simulink model "chibiOS_Config_Test_PAL"  (R2015b)
settings: Solver=FixedStepDiscrete  SolverMode=MultiTasking  StartTime=0.0  StopTime=10.0  RelTol=1e-3
undefined symbols (not defined in the file or in its folder): chSysHalt, STM32_DMA_STREAM_ID
libraries: lib_ChibiOS x3
settings Model: Creator=freyjed  LastModifiedBy=C3038028
settings DataIOCC: LimitDataPoints=off  SaveFormat=Array  SaveOutput=off  SignalLogging=off  DSMLogging=off  SaveTime=off
settings OptimizationCC: BlockReduction=off  ConditionallyExecuteInputs=off  BufferReuse=off  ExpressionDepthLimit=2147483647  OptimizeModelRefInitCode=on  LifeSpan=1
settings DebuggingCC: UnderspecifiedInitializationDetection=Classic  MergeDetectMultiDrivingBlocksExec=none  SolverPrmCheckMsg=warning  StateNameClashWarn=warning
settings HardwareCC: ProdBitPerPointer=32  ProdLargestAtomicInteger=Integer  ProdWordSize=32  ProdHWDeviceType=STMicroelectronics->STM32F4xx 32-bit Cortex-M4  TargetLargestAtomicInteger=Integer  TargetLargestAtomicFloat=Float  TargetIntDivRoundTo=Zero  TargetEndianess=LittleEndian  TargetHWDeviceType=ChibiOS->ChibiOS
settings ModelReferenceCC: UpdateModelReferenceTargets=Force
settings RTWCC: SystemTargetFile=ChibiOS.tlc  GenCodeOnly=on  TemplateMakefile=ChibiOS.tmf  Description=ChibiOS/RT (Embedded RTOS Target)  RetainRTWFile=on  IncludeHyperlinkInReport=on
settings CodeAppCC: ForceParamTrailComments=on  IgnoreCustomStorageClasses=off  OperatorAnnotations=on  SimulinkDataObjDesc=on  SFDataObjDesc=on  MATLABFcnDesc=on  CustomSymbolStrType=$N$R$M  DefineNamingRule=UpperCase  InsertBlockDesc=on  MATLABSourceComments=on  InternalIdentifier=Classic  ReqsInCode=on
settings STFCustomTargetCC: ModelReferenceCompliant=off  ConcurrentExecutionCompliant=off  IncludeMdlTerminateFcn=off  GeneratePreprocessorConditionals=Use local settings  CombineOutputUpdateFcns=on  ERTCustomFileBanners=on  SupportContinuousTime=off  SupportNonInlinedSFcns=off  ParenthesesLevel=Maximum  MATLABClassNameForMDSCustomization=Simulink.SoftwareTarget.ERTCustomization  CPPClassGenCompliant=off  GRTInterface=off  SystemTargetFile=ChibiOS.tlc
settings ERTTargetCC: ModelReferenceCompliant=off  ParMdlRefBuildCompliant=off  CompOptLevelCompliant=off  ConcurrentExecutionCompliant=off  IncludeMdlTerminateFcn=off  ERTFirstTimeCompliant=off  ParenthesesLevel=Maximum  ModelStepFunctionPrototypeControlCompliant=off  CPPClassGenCompliant=off  UseToolchainInfoCompliant=off  ERTSrcFileBannerTemplate=chibiOS_sourceFileTemplate.cgt  ERTHdrFileBannerTemplate=chibiOS_sourceFileTemplate.cgt  ERTDataSrcFileTemplate=chibiOS_sourceFileTemplate.cgt  ERTDataHdrFileTemplate=chibiOS_sourceFileTemplate.cgt  ERTCustomFileTemplate=chibiOS_customRoutineProcess.tlc  PreserveExpressionOrder=on  PreserveIfCondition=on  ConvertIfToSwitch=on
settings ConfigComp: CovModelRefEnable=Off

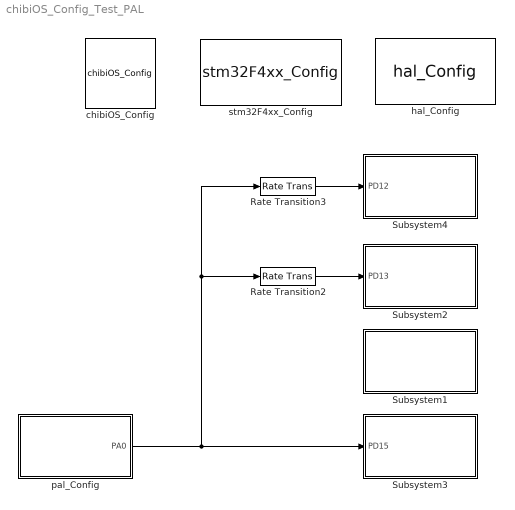
== system chibiOS_Config_Test_PAL ==
  Rate Transition2 : RateTransition
  Rate Transition3 : RateTransition
  Subsystem1 : Subsystem  mask(pal_Config){portName=D, pin0=Disabled, pin1=Disabled, pin2=Disabled, pin3=Disabled, pin4=Disabled, pin5=Disabled, pin6=Disabled, pin7=Disabled, pin8=Disabled, pin9=Disabled, pin10=Disabled, pin11=Disabled, pin12=Disabled, pin13=Disabled, pin14=Toggle, pin15=Disabled, pal_Ts=.9}
      mask prompts: portName "Port"; pin0 "Pin 0"; pin1 "Pin 1"; pin2 "Pin 2"; pin3 "Pin 3"; pin4 "Pin 4"; pin5 "Pin 5"; pin6 "Pin 6"; pin7 "Pin 7"; pin8 "Pin 8"; pin9 "Pin 9"; pin10 "Pin 10"; pin11 "Pin 11"; pin12 "Pin 12"; pin13 "Pin 13"; pin14 "Pin 14"; pin15 "Pin 15"; pal_Ts "Sample Time (-1 for inherited)"
      mask TypeOptions portName: A | B | C | D | E | F | G | H | I
      mask Callback portName: pal_Config_Callback(gcb)
      mask TypeOptions pin0: Disabled | Input - No Pull | Input - Pull Up | Input - Pull Down | Output - Open Drain | Output - Push Pull | Toggle
      mask Callback pin0: pal_Config_Callback(gcb)
      mask TypeOptions pin1: Disabled | Input - No Pull | Input - Pull Up | Input - Pull Down | Output - Open Drain | Output - Push Pull | Toggle
      mask Callback pin1: pal_Config_Callback(gcb)
      mask TypeOptions pin2: Disabled | Input - No Pull | Input - Pull Up | Input - Pull Down | Output - Open Drain | Output - Push Pull | Toggle
      mask Callback pin2: pal_Config_Callback(gcb)
      mask TypeOptions pin3: Disabled | Input - No Pull | Input - Pull Up | Input - Pull Down | Output - Open Drain | Output - Push Pull | Toggle
      mask Callback pin3: pal_Config_Callback(gcb)
      mask TypeOptions pin4: Disabled | Input - No Pull | Input - Pull Up | Input - Pull Down | Output - Open Drain | Output - Push Pull | Toggle
      mask Callback pin4: pal_Config_Callback(gcb)
      mask TypeOptions pin5: Disabled | Input - No Pull | Input - Pull Up | Input - Pull Down | Output - Open Drain | Output - Push Pull | Toggle
      mask Callback pin5: pal_Config_Callback(gcb)
      mask TypeOptions pin6: Disabled | Input - No Pull | Input - Pull Up | Input - Pull Down | Output - Open Drain | Output - Push Pull | Toggle
      mask Callback pin6: pal_Config_Callback(gcb)
      mask TypeOptions pin7: Disabled | Input - No Pull | Input - Pull Up | Input - Pull Down | Output - Open Drain | Output - Push Pull | Toggle
      mask Callback pin7: pal_Config_Callback(gcb)
      mask TypeOptions pin8: Disabled | Input - No Pull | Input - Pull Up | Input - Pull Down | Output - Open Drain | Output - Push Pull | Toggle
      mask Callback pin8: pal_Config_Callback(gcb)
      mask TypeOptions pin9: Disabled | Input - No Pull | Input - Pull Up | Input - Pull Down | Output - Open Drain | Output - Push Pull | Toggle
      mask Callback pin9: pal_Config_Callback(gcb)
      mask TypeOptions pin10: Disabled | Input - No Pull | Input - Pull Up | Input - Pull Down | Output - Open Drain | Output - Push Pull | Toggle
      mask Callback pin10: pal_Config_Callback(gcb)
      mask TypeOptions pin11: Disabled | Input - No Pull | Input - Pull Up | Input - Pull Down | Output - Open Drain | Output - Push Pull | Toggle
      mask Callback pin11: pal_Config_Callback(gcb)
      mask TypeOptions pin12: Disabled | Input - No Pull | Input - Pull Up | Input - Pull Down | Output - Open Drain | Output - Push Pull | Toggle
      mask Callback pin12: pal_Config_Callback(gcb)
      mask TypeOptions pin13: Disabled | Input - No Pull | Input - Pull Up | Input - Pull Down | Output - Open Drain | Output - Push Pull | Toggle
      mask Callback pin13: pal_Config_Callback(gcb)
      mask TypeOptions pin14: Disabled | Input - No Pull | Input - Pull Up | Input - Pull Down | Output - Open Drain | Output - Push Pull | Toggle
      mask Callback pin14: pal_Config_Callback(gcb)
      mask TypeOptions pin15: Disabled | Input - No Pull | Input - Pull Up | Input - Pull Down | Output - Open Drain | Output - Push Pull | Toggle
      mask Callback pin15: pal_Config_Callback(gcb)
  Subsystem2 : Subsystem  mask(pal_Config){portName=D, pin0=Disabled, pin1=Disabled, pin2=Disabled, pin3=Disabled, pin4=Disabled, pin5=Disabled, pin6=Disabled, pin7=Disabled, pin8=Disabled, pin9=Disabled, pin10=Disabled, pin11=Disabled, pin12=Disabled, pin13=Output - Push Pull, pin14=Disabled, pin15=Disabled, pal_Ts=.015*6}
      mask prompts: portName "Port"; pin0 "Pin 0"; pin1 "Pin 1"; pin2 "Pin 2"; pin3 "Pin 3"; pin4 "Pin 4"; pin5 "Pin 5"; pin6 "Pin 6"; pin7 "Pin 7"; pin8 "Pin 8"; pin9 "Pin 9"; pin10 "Pin 10"; pin11 "Pin 11"; pin12 "Pin 12"; pin13 "Pin 13"; pin14 "Pin 14"; pin15 "Pin 15"; pal_Ts "Sample Time (-1 for inherited)"
      mask TypeOptions portName: A | B | C | D | E | F | G | H | I
      mask Callback portName: pal_Config_Callback(gcb)
      mask TypeOptions pin0: Disabled | Input - No Pull | Input - Pull Up | Input - Pull Down | Output - Open Drain | Output - Push Pull | Toggle
      mask Callback pin0: pal_Config_Callback(gcb)
      mask TypeOptions pin1: Disabled | Input - No Pull | Input - Pull Up | Input - Pull Down | Output - Open Drain | Output - Push Pull | Toggle
      mask Callback pin1: pal_Config_Callback(gcb)
      mask TypeOptions pin2: Disabled | Input - No Pull | Input - Pull Up | Input - Pull Down | Output - Open Drain | Output - Push Pull | Toggle
      mask Callback pin2: pal_Config_Callback(gcb)
      mask TypeOptions pin3: Disabled | Input - No Pull | Input - Pull Up | Input - Pull Down | Output - Open Drain | Output - Push Pull | Toggle
      mask Callback pin3: pal_Config_Callback(gcb)
      mask TypeOptions pin4: Disabled | Input - No Pull | Input - Pull Up | Input - Pull Down | Output - Open Drain | Output - Push Pull | Toggle
      mask Callback pin4: pal_Config_Callback(gcb)
      mask TypeOptions pin5: Disabled | Input - No Pull | Input - Pull Up | Input - Pull Down | Output - Open Drain | Output - Push Pull | Toggle
      mask Callback pin5: pal_Config_Callback(gcb)
      mask TypeOptions pin6: Disabled | Input - No Pull | Input - Pull Up | Input - Pull Down | Output - Open Drain | Output - Push Pull | Toggle
      mask Callback pin6: pal_Config_Callback(gcb)
      mask TypeOptions pin7: Disabled | Input - No Pull | Input - Pull Up | Input - Pull Down | Output - Open Drain | Output - Push Pull | Toggle
      mask Callback pin7: pal_Config_Callback(gcb)
      mask TypeOptions pin8: Disabled | Input - No Pull | Input - Pull Up | Input - Pull Down | Output - Open Drain | Output - Push Pull | Toggle
      mask Callback pin8: pal_Config_Callback(gcb)
      mask TypeOptions pin9: Disabled | Input - No Pull | Input - Pull Up | Input - Pull Down | Output - Open Drain | Output - Push Pull | Toggle
      mask Callback pin9: pal_Config_Callback(gcb)
      mask TypeOptions pin10: Disabled | Input - No Pull | Input - Pull Up | Input - Pull Down | Output - Open Drain | Output - Push Pull | Toggle
      mask Callback pin10: pal_Config_Callback(gcb)
      mask TypeOptions pin11: Disabled | Input - No Pull | Input - Pull Up | Input - Pull Down | Output - Open Drain | Output - Push Pull | Toggle
      mask Callback pin11: pal_Config_Callback(gcb)
      mask TypeOptions pin12: Disabled | Input - No Pull | Input - Pull Up | Input - Pull Down | Output - Open Drain | Output - Push Pull | Toggle
      mask Callback pin12: pal_Config_Callback(gcb)
      mask TypeOptions pin13: Disabled | Input - No Pull | Input - Pull Up | Input - Pull Down | Output - Open Drain | Output - Push Pull | Toggle
      mask Callback pin13: pal_Config_Callback(gcb)
      mask TypeOptions pin14: Disabled | Input - No Pull | Input - Pull Up | Input - Pull Down | Output - Open Drain | Output - Push Pull | Toggle
      mask Callback pin14: pal_Config_Callback(gcb)
      mask TypeOptions pin15: Disabled | Input - No Pull | Input - Pull Up | Input - Pull Down | Output - Open Drain | Output - Push Pull | Toggle
      mask Callback pin15: pal_Config_Callback(gcb)
  Subsystem3 : Subsystem  mask(pal_Config){portName=D, pin0=Disabled, pin1=Disabled, pin2=Disabled, pin3=Disabled, pin4=Disabled, pin5=Disabled, pin6=Disabled, pin7=Disabled, pin8=Disabled, pin9=Disabled, pin10=Disabled, pin11=Disabled, pin12=Disabled, pin13=Disabled, pin14=Disabled, pin15=Output - Push Pull, pal_Ts=0.015}
      mask prompts: portName "Port"; pin0 "Pin 0"; pin1 "Pin 1"; pin2 "Pin 2"; pin3 "Pin 3"; pin4 "Pin 4"; pin5 "Pin 5"; pin6 "Pin 6"; pin7 "Pin 7"; pin8 "Pin 8"; pin9 "Pin 9"; pin10 "Pin 10"; pin11 "Pin 11"; pin12 "Pin 12"; pin13 "Pin 13"; pin14 "Pin 14"; pin15 "Pin 15"; pal_Ts "Sample Time (-1 for inherited)"
      mask TypeOptions portName: A | B | C | D | E | F | G | H | I
      mask Callback portName: pal_Config_Callback(gcb)
      mask TypeOptions pin0: Disabled | Input - No Pull | Input - Pull Up | Input - Pull Down | Output - Open Drain | Output - Push Pull | Toggle
      mask Callback pin0: pal_Config_Callback(gcb)
      mask TypeOptions pin1: Disabled | Input - No Pull | Input - Pull Up | Input - Pull Down | Output - Open Drain | Output - Push Pull | Toggle
      mask Callback pin1: pal_Config_Callback(gcb)
      mask TypeOptions pin2: Disabled | Input - No Pull | Input - Pull Up | Input - Pull Down | Output - Open Drain | Output - Push Pull | Toggle
      mask Callback pin2: pal_Config_Callback(gcb)
      mask TypeOptions pin3: Disabled | Input - No Pull | Input - Pull Up | Input - Pull Down | Output - Open Drain | Output - Push Pull | Toggle
      mask Callback pin3: pal_Config_Callback(gcb)
      mask TypeOptions pin4: Disabled | Input - No Pull | Input - Pull Up | Input - Pull Down | Output - Open Drain | Output - Push Pull | Toggle
      mask Callback pin4: pal_Config_Callback(gcb)
      mask TypeOptions pin5: Disabled | Input - No Pull | Input - Pull Up | Input - Pull Down | Output - Open Drain | Output - Push Pull | Toggle
      mask Callback pin5: pal_Config_Callback(gcb)
      mask TypeOptions pin6: Disabled | Input - No Pull | Input - Pull Up | Input - Pull Down | Output - Open Drain | Output - Push Pull | Toggle
      mask Callback pin6: pal_Config_Callback(gcb)
      mask TypeOptions pin7: Disabled | Input - No Pull | Input - Pull Up | Input - Pull Down | Output - Open Drain | Output - Push Pull | Toggle
      mask Callback pin7: pal_Config_Callback(gcb)
      mask TypeOptions pin8: Disabled | Input - No Pull | Input - Pull Up | Input - Pull Down | Output - Open Drain | Output - Push Pull | Toggle
      mask Callback pin8: pal_Config_Callback(gcb)
      mask TypeOptions pin9: Disabled | Input - No Pull | Input - Pull Up | Input - Pull Down | Output - Open Drain | Output - Push Pull | Toggle
      mask Callback pin9: pal_Config_Callback(gcb)
      mask TypeOptions pin10: Disabled | Input - No Pull | Input - Pull Up | Input - Pull Down | Output - Open Drain | Output - Push Pull | Toggle
      mask Callback pin10: pal_Config_Callback(gcb)
      mask TypeOptions pin11: Disabled | Input - No Pull | Input - Pull Up | Input - Pull Down | Output - Open Drain | Output - Push Pull | Toggle
      mask Callback pin11: pal_Config_Callback(gcb)
      mask TypeOptions pin12: Disabled | Input - No Pull | Input - Pull Up | Input - Pull Down | Output - Open Drain | Output - Push Pull | Toggle
      mask Callback pin12: pal_Config_Callback(gcb)
      mask TypeOptions pin13: Disabled | Input - No Pull | Input - Pull Up | Input - Pull Down | Output - Open Drain | Output - Push Pull | Toggle
      mask Callback pin13: pal_Config_Callback(gcb)
      mask TypeOptions pin14: Disabled | Input - No Pull | Input - Pull Up | Input - Pull Down | Output - Open Drain | Output - Push Pull | Toggle
      mask Callback pin14: pal_Config_Callback(gcb)
      mask TypeOptions pin15: Disabled | Input - No Pull | Input - Pull Up | Input - Pull Down | Output - Open Drain | Output - Push Pull | Toggle
      mask Callback pin15: pal_Config_Callback(gcb)
  Subsystem4 : Subsystem  mask(pal_Config){portName=D, pin0=Disabled, pin1=Disabled, pin2=Disabled, pin3=Disabled, pin4=Disabled, pin5=Disabled, pin6=Disabled, pin7=Disabled, pin8=Disabled, pin9=Disabled, pin10=Disabled, pin11=Disabled, pin12=Output - Push Pull, pin13=Disabled, pin14=Disabled, pin15=Disabled, pal_Ts=.015*4}
      mask prompts: portName "Port"; pin0 "Pin 0"; pin1 "Pin 1"; pin2 "Pin 2"; pin3 "Pin 3"; pin4 "Pin 4"; pin5 "Pin 5"; pin6 "Pin 6"; pin7 "Pin 7"; pin8 "Pin 8"; pin9 "Pin 9"; pin10 "Pin 10"; pin11 "Pin 11"; pin12 "Pin 12"; pin13 "Pin 13"; pin14 "Pin 14"; pin15 "Pin 15"; pal_Ts "Sample Time (-1 for inherited)"
      mask TypeOptions portName: A | B | C | D | E | F | G | H | I
      mask Callback portName: pal_Config_Callback(gcb)
      mask TypeOptions pin0: Disabled | Input - No Pull | Input - Pull Up | Input - Pull Down | Output - Open Drain | Output - Push Pull | Toggle
      mask Callback pin0: pal_Config_Callback(gcb)
      mask TypeOptions pin1: Disabled | Input - No Pull | Input - Pull Up | Input - Pull Down | Output - Open Drain | Output - Push Pull | Toggle
      mask Callback pin1: pal_Config_Callback(gcb)
      mask TypeOptions pin2: Disabled | Input - No Pull | Input - Pull Up | Input - Pull Down | Output - Open Drain | Output - Push Pull | Toggle
      mask Callback pin2: pal_Config_Callback(gcb)
      mask TypeOptions pin3: Disabled | Input - No Pull | Input - Pull Up | Input - Pull Down | Output - Open Drain | Output - Push Pull | Toggle
      mask Callback pin3: pal_Config_Callback(gcb)
      mask TypeOptions pin4: Disabled | Input - No Pull | Input - Pull Up | Input - Pull Down | Output - Open Drain | Output - Push Pull | Toggle
      mask Callback pin4: pal_Config_Callback(gcb)
      mask TypeOptions pin5: Disabled | Input - No Pull | Input - Pull Up | Input - Pull Down | Output - Open Drain | Output - Push Pull | Toggle
      mask Callback pin5: pal_Config_Callback(gcb)
      mask TypeOptions pin6: Disabled | Input - No Pull | Input - Pull Up | Input - Pull Down | Output - Open Drain | Output - Push Pull | Toggle
      mask Callback pin6: pal_Config_Callback(gcb)
      mask TypeOptions pin7: Disabled | Input - No Pull | Input - Pull Up | Input - Pull Down | Output - Open Drain | Output - Push Pull | Toggle
      mask Callback pin7: pal_Config_Callback(gcb)
      mask TypeOptions pin8: Disabled | Input - No Pull | Input - Pull Up | Input - Pull Down | Output - Open Drain | Output - Push Pull | Toggle
      mask Callback pin8: pal_Config_Callback(gcb)
      mask TypeOptions pin9: Disabled | Input - No Pull | Input - Pull Up | Input - Pull Down | Output - Open Drain | Output - Push Pull | Toggle
      mask Callback pin9: pal_Config_Callback(gcb)
      mask TypeOptions pin10: Disabled | Input - No Pull | Input - Pull Up | Input - Pull Down | Output - Open Drain | Output - Push Pull | Toggle
      mask Callback pin10: pal_Config_Callback(gcb)
      mask TypeOptions pin11: Disabled | Input - No Pull | Input - Pull Up | Input - Pull Down | Output - Open Drain | Output - Push Pull | Toggle
      mask Callback pin11: pal_Config_Callback(gcb)
      mask TypeOptions pin12: Disabled | Input - No Pull | Input - Pull Up | Input - Pull Down | Output - Open Drain | Output - Push Pull | Toggle
      mask Callback pin12: pal_Config_Callback(gcb)
      mask TypeOptions pin13: Disabled | Input - No Pull | Input - Pull Up | Input - Pull Down | Output - Open Drain | Output - Push Pull | Toggle
      mask Callback pin13: pal_Config_Callback(gcb)
      mask TypeOptions pin14: Disabled | Input - No Pull | Input - Pull Up | Input - Pull Down | Output - Open Drain | Output - Push Pull | Toggle
      mask Callback pin14: pal_Config_Callback(gcb)
      mask TypeOptions pin15: Disabled | Input - No Pull | Input - Pull Up | Input - Pull Down | Output - Open Drain | Output - Push Pull | Toggle
      mask Callback pin15: pal_Config_Callback(gcb)
  chibiOS_Config : lib_ChibiOS/chibiOS_Config  CH_FREQUENCY=1000  CH_TIME_QUANTUM=20  CH_MEMCORE_SIZE=0  CH_NO_IDLE_THREAD=off  CH_OPTIMIZE_SPEED=on  CH_USE_REGISTRY=on  CH_USE_WAITEXIT=on  CH_USE_SEMAPHORES=on  CH_USE_SEMAPHORES_PRIORITY=off  CH_USE_SEMSW=on  CH_USE_MUTEXES=on  CH_USE_CONDVARS=on  CH_USE_CONDVARS_TIMEOUT=on  CH_USE_EVENTS=on  CH_USE_EVENTS_TIMEOUT=on  CH_USE_MESSAGES=on  CH_USE_MESSAGES_PRIORITY=off  CH_USE_MAILBOXES=on  CH_USE_QUEUES=on  CH_USE_MEMCORE=on  CH_USE_HEAP=on  CH_USE_MALLOC_HEAP=off  CH_USE_MEMPOOLS=on  CH_USE_DYNAMIC=on  CH_DBG_SYSTEM_STATE_CHECK=on  CH_DBG_ENABLE_CHECKS=on  CH_DBG_ENABLE_ASSERTS=on  CH_DBG_ENABLE_TRACE=on  CH_DBG_ENABLE_STACK_CHECK=on  CH_DBG_FILL_THREADS=on  CH_DBG_THREADS_PROFILING=on
  hal_Config : lib_ChibiOS/hal_Config  HAL_USE_TM=on  HAL_USE_PAL=on  HAL_USE_ADC=off  HAL_USE_CAN=off  HAL_USE_EXT=off  HAL_USE_GPT=off  HAL_USE_I2C=off  HAL_USE_ICU=off  HAL_USE_MAC=off  HAL_USE_MMC_SPI=off  HAL_USE_PWM=on  HAL_USE_RTC=off  HAL_USE_SDC=off  HAL_USE_SERIAL=off  HAL_USE_SERIAL_USB=off  HAL_USE_SPI=on  HAL_USE_UART=off  HAL_USE_USB=off  ADC_USE_WAIT=on  ADC_USE_MUTUAL_EXCLUSION=on  CAN_USE_SLEEP_MODE=on  I2C_USE_MUTUAL_EXCLUSION=on  MAC_USE_ZERO_COPY=off  MAC_USE_EVENTS=on  MMC_NICE_WAITING=on  SDC_INIT_RETRY=100  SDC_MMC_SUPPORT=off  SDC_NICE_WAITING=on  SERIAL_DEFAULT_BITRATE=38400  SERIAL_BUFFERS_SIZE=16  SPI_USE_WAIT=on  SPI_USE_MUTUAL_EXCLUSION=off
  pal_Config : Subsystem  AncestorBlock=lib_ChibiOS/pal_Config  mask(pal_Config){portName=A, pin0=Input - No Pull, pin1=Disabled, pin2=Disabled, pin3=Disabled, pin4=Disabled, pin5=Disabled, pin6=Disabled, pin7=Disabled, pin8=Disabled, pin9=Disabled, pin10=Disabled, pin11=Disabled, pin12=Disabled, pin13=Disabled, pin14=Disabled, pin15=Disabled, pal_Ts=0.015}
      mask prompts: portName "Port"; pin0 "Pin 0"; pin1 "Pin 1"; pin2 "Pin 2"; pin3 "Pin 3"; pin4 "Pin 4"; pin5 "Pin 5"; pin6 "Pin 6"; pin7 "Pin 7"; pin8 "Pin 8"; pin9 "Pin 9"; pin10 "Pin 10"; pin11 "Pin 11"; pin12 "Pin 12"; pin13 "Pin 13"; pin14 "Pin 14"; pin15 "Pin 15"; pal_Ts "Sample Time (-1 for inherited)"
      mask TypeOptions portName: A | B | C | D | E | F | G | H | I
      mask Callback portName: pal_Config_Callback(gcb)
      mask TypeOptions pin0: Disabled | Input - No Pull | Input - Pull Up | Input - Pull Down | Output - Open Drain | Output - Push Pull | Toggle
      mask Callback pin0: pal_Config_Callback(gcb)
      mask TypeOptions pin1: Disabled | Input - No Pull | Input - Pull Up | Input - Pull Down | Output - Open Drain | Output - Push Pull | Toggle
      mask Callback pin1: pal_Config_Callback(gcb)
      mask TypeOptions pin2: Disabled | Input - No Pull | Input - Pull Up | Input - Pull Down | Output - Open Drain | Output - Push Pull | Toggle
      mask Callback pin2: pal_Config_Callback(gcb)
      mask TypeOptions pin3: Disabled | Input - No Pull | Input - Pull Up | Input - Pull Down | Output - Open Drain | Output - Push Pull | Toggle
      mask Callback pin3: pal_Config_Callback(gcb)
      mask TypeOptions pin4: Disabled | Input - No Pull | Input - Pull Up | Input - Pull Down | Output - Open Drain | Output - Push Pull | Toggle
      mask Callback pin4: pal_Config_Callback(gcb)
      mask TypeOptions pin5: Disabled | Input - No Pull | Input - Pull Up | Input - Pull Down | Output - Open Drain | Output - Push Pull | Toggle
      mask Callback pin5: pal_Config_Callback(gcb)
      mask TypeOptions pin6: Disabled | Input - No Pull | Input - Pull Up | Input - Pull Down | Output - Open Drain | Output - Push Pull | Toggle
      mask Callback pin6: pal_Config_Callback(gcb)
      mask TypeOptions pin7: Disabled | Input - No Pull | Input - Pull Up | Input - Pull Down | Output - Open Drain | Output - Push Pull | Toggle
      mask Callback pin7: pal_Config_Callback(gcb)
      mask TypeOptions pin8: Disabled | Input - No Pull | Input - Pull Up | Input - Pull Down | Output - Open Drain | Output - Push Pull | Toggle
      mask Callback pin8: pal_Config_Callback(gcb)
      mask TypeOptions pin9: Disabled | Input - No Pull | Input - Pull Up | Input - Pull Down | Output - Open Drain | Output - Push Pull | Toggle
      mask Callback pin9: pal_Config_Callback(gcb)
      mask TypeOptions pin10: Disabled | Input - No Pull | Input - Pull Up | Input - Pull Down | Output - Open Drain | Output - Push Pull | Toggle
      mask Callback pin10: pal_Config_Callback(gcb)
      mask TypeOptions pin11: Disabled | Input - No Pull | Input - Pull Up | Input - Pull Down | Output - Open Drain | Output - Push Pull | Toggle
      mask Callback pin11: pal_Config_Callback(gcb)
      mask TypeOptions pin12: Disabled | Input - No Pull | Input - Pull Up | Input - Pull Down | Output - Open Drain | Output - Push Pull | Toggle
      mask Callback pin12: pal_Config_Callback(gcb)
      mask TypeOptions pin13: Disabled | Input - No Pull | Input - Pull Up | Input - Pull Down | Output - Open Drain | Output - Push Pull | Toggle
      mask Callback pin13: pal_Config_Callback(gcb)
      mask TypeOptions pin14: Disabled | Input - No Pull | Input - Pull Up | Input - Pull Down | Output - Open Drain | Output - Push Pull | Toggle
      mask Callback pin14: pal_Config_Callback(gcb)
      mask TypeOptions pin15: Disabled | Input - No Pull | Input - Pull Up | Input - Pull Down | Output - Open Drain | Output - Push Pull | Toggle
      mask Callback pin15: pal_Config_Callback(gcb)
  stm32F4xx_Config : lib_ChibiOS/stm32F4xx_Config  STM32_NO_INIT=off  STM32_HSI_ENABLED=on  STM32_LSI_ENABLED=on  STM32_HSE_ENABLED=on  STM32_LSE_ENABLED=off  STM32_CLOCK48_REQUIRED=on  STM32_SW=Phase locked Loop (PLL)  STM32_PLLSRC=External High Speed Clock (HSE)  STM32_PLLM_VALUE=8  STM32_PLLN_VALUE=336  STM32_PLLP_VALUE=2  STM32_PLLQ_VALUE=7  STM32_HPRE=1  STM32_PPRE1=4  STM32_PPRE2=2  STM32_RTCSEL=LSI  STM32_RTCPRE_VALUE=8  STM32_MCO1SEL=HSI clock on MCO1 pin  STM32_MCO1PRE=1  STM32_MCO2SEL=SYSCLK clock on MCO2 pin  STM32_MCO2PRE=5  STM32_I2SSRC=CKIN  STM32_PLLI2SN_VALUE=192  STM32_PLLI2SR_VALUE=5  STM32_VOS=STM32_VOS_HIGH  STM32_PVD_ENABLE=off  STM32_PLS=Level 0: 214/204 mV  STM32_ADC_ADCPRE=2  STM32_ADC_IRQ_PRIORITY=6  STM32_ADC_USE_ADC1=off  STM32_ADC_ADC1_DMA_STREAM=STM32_DMA_STREAM_ID(2, 4)  STM32_ADC_ADC1_DMA_PRIORITY=2  STM32_ADC_ADC1_DMA_IRQ_PRIORITY=6  STM32_ADC_USE_ADC2=off  STM32_ADC_ADC2_DMA_STREAM=STM32_DMA_STREAM_ID(2, 3)  STM32_ADC_ADC2_DMA_PRIORITY=2  STM32_ADC_ADC2_DMA_IRQ_PRIORITY=6  STM32_ADC_USE_ADC3=off  STM32_ADC_ADC3_DMA_STREAM=STM32_DMA_STREAM_ID(2, 1)  STM32_ADC_ADC3_DMA_PRIORITY=2  STM32_ADC_ADC3_DMA_IRQ_PRIORITY=6  STM32_CAN_USE_CAN1=off  STM32_CAN_CAN1_IRQ_PRIORITY=11  STM32_CAN_USE_CAN2=off  STM32_CAN_CAN2_IRQ_PRIORITY=11  STM32_EXT_EXTI0_IRQ_PRIORITY=10  STM32_EXT_EXTI1_IRQ_PRIORITY=10  STM32_EXT_EXTI2_IRQ_PRIORITY=10  STM32_EXT_EXTI3_IRQ_PRIORITY=10  STM32_EXT_EXTI4_IRQ_PRIORITY=10  STM32_EXT_EXTI5_9_IRQ_PRIORITY=10  STM32_EXT_EXTI10_15_IRQ_PRIORITY=10  STM32_EXT_EXTI16_IRQ_PRIORITY=10  STM32_EXT_EXTI17_IRQ_PRIORITY=1  STM32_EXT_EXTI18_IRQ_PRIORITY=10  STM32_EXT_EXTI19_IRQ_PRIORITY=10  STM32_EXT_EXTI20_IRQ_PRIORITY=10  STM32_EXT_EXTI21_IRQ_PRIORITY=1  STM32_EXT_EXTI22_IRQ_PRIORITY=1  STM32_GPT_USE_TIM1=off  STM32_GPT_TIM1_IRQ_PRIORITY=9  STM32_GPT_USE_TIM2=off  STM32_GPT_TIM2_IRQ_PRIORITY=9  STM32_GPT_USE_TIM3=off  STM32_GPT_TIM3_IRQ_PRIORITY=9  STM32_GPT_USE_TIM4=off  STM32_GPT_TIM4_IRQ_PRIORITY=9  STM32_GPT_USE_TIM5=off  STM32_GPT_TIM5_IRQ_PRIORITY=9  STM32_GPT_USE_TIM6=off  STM32_GPT_TIM6_IRQ_PRIORITY=9  STM32_GPT_USE_TIM7=off  STM32_GPT_TIM7_IRQ_PRIORITY=9  STM32_GPT_USE_TIM8=off  STM32_GPT_TIM8_IRQ_PRIORITY=9  STM32_GPT_USE_TIM9=off  STM32_GPT_TIM9_IRQ_PRIORITY=9  STM32_GPT_USE_TIM11=off  STM32_GPT_TIM11_IRQ_PRIORITY=9  STM32_GPT_USE_TIM12=off  STM32_GPT_TIM12_IRQ_PRIORITY=9  STM32_GPT_USE_TIM14=off  STM32_GPT_TIM14_IRQ_PRIORITY=9  STM32_I2C_USE_I2C1=off  STM32_I2C_I2C1_RX_DMA_STREAM=STM32_DMA_STREAM_ID(1, 0)  STM32_I2C_I2C1_TX_DMA_STREAM=STM32_DMA_STREAM_ID(1, 6)  STM32_I2C_I2C1_IRQ_PRIORITY=11  STM32_I2C_I2C1_DMA_PRIORITY=3  STM32_I2C_I2C1_DMA_ERROR_HOOK=chSysHalt()  STM32_I2C_USE_I2C2=off  STM32_I2C_I2C2_RX_DMA_STREAM=STM32_DMA_STREAM_ID(1, 2)  STM32_I2C_I2C2_TX_DMA_STREAM=STM32_DMA_STREAM_ID(1, 7)  STM32_I2C_I2C2_IRQ_PRIORITY=11  STM32_I2C_I2C2_DMA_PRIORITY=3  STM32_I2C_I2C2_DMA_ERROR_HOOK=chSysHalt()  STM32_I2C_USE_I2C3=off  STM32_I2C_I2C3_RX_DMA_STREAM=STM32_DMA_STREAM_ID(1, 2)  STM32_I2C_I2C3_TX_DMA_STREAM=STM32_DMA_STREAM_ID(1, 4)  STM32_I2C_I2C3_IRQ_PRIORITY=11  STM32_I2C_I2C3_DMA_PRIORITY=3  STM32_I2C_I2C3_DMA_ERROR_HOOK=chSysHalt()  STM32_ICU_USE_TIM1=off  STM32_ICU_TIM1_IRQ_PRIORITY=9  STM32_ICU_USE_TIM2=off  STM32_ICU_TIM2_IRQ_PRIORITY=9  STM32_ICU_USE_TIM3=off  STM32_ICU_TIM3_IRQ_PRIORITY=9  STM32_ICU_USE_TIM4=off  STM32_ICU_TIM4_IRQ_PRIORITY=9  STM32_ICU_USE_TIM5=off  STM32_ICU_TIM5_IRQ_PRIORITY=9  STM32_ICU_USE_TIM8=off  STM32_ICU_TIM8_IRQ_PRIORITY=9  STM32_ICU_USE_TIM9=off  STM32_ICU_TIM9_IRQ_PRIORITY=9  STM32_MAC_TRANSMIT_BUFFERS=2  STM32_MAC_RECEIVE_BUFFERS=4  STM32_MAC_BUFFERS_SIZE=1522  STM32_MAC_PHY_TIMEOUT=100  STM32_MAC_ETH1_CHANGE_PHY_STATE=on  STM32_MAC_ETH1_IRQ_PRIORITY=13  STM32_MAC_IP_CHECKSUM_OFFLOAD=0  STM32_PWM_USE_ADVANCED=off  STM32_PWM_USE_TIM1=off  STM32_PWM_TIM1_IRQ_PRIORITY=9  STM32_PWM_USE_TIM2=off  STM32_PWM_TIM2_IRQ_PRIORITY=9  STM32_PWM_USE_TIM3=on  STM32_PWM_TIM3_IRQ_PRIORITY=9  STM32_PWM_USE_TIM4=on  STM32_PWM_TIM4_IRQ_PRIORITY=9  STM32_PWM_USE_TIM5=off  STM32_PWM_TIM5_IRQ_PRIORITY=9  STM32_PWM_USE_TIM8=off  STM32_PWM_TIM8_IRQ_PRIORITY=9  STM32_PWM_USE_TIM9=off  STM32_PWM_TIM9_IRQ_PRIORITY=9  STM32_SERIAL_USE_USART1=off  STM32_SERIAL_USART1_PRIORITY=4  STM32_SERIAL_USE_USART2=off  STM32_SERIAL_USART2_PRIORITY=4  STM32_SERIAL_USE_USART3=off  STM32_SERIAL_USART3_PRIORITY=4  STM32_SERIAL_USE_UART4=off  STM32_SERIAL_UART4_PRIORITY=4  STM32_SERIAL_USE_UART5=off  STM32_SERIAL_UART5_PRIORITY=4  STM32_SERIAL_USE_USART6=off  STM32_SERIAL_USART6_PRIORITY=4  STM32_SPI_USE_SPI1=off  STM32_SPI_SPI1_RX_DMA_STREAM=STM32_DMA_STREAM_ID(2,0)  STM32_SPI_SPI1_TX_DMA_STREAM=STM32_DMA_STREAM_ID(2,3)  STM32_SPI_SPI1_DMA_PRIORITY=2  STM32_SPI_SPI1_IRQ_PRIORITY=6  STM32_SPI_USE_SPI2=off  STM32_SPI_SPI2_RX_DMA_STREAM=STM32_DMA_STREAM_ID(1,3)  STM32_SPI_SPI2_TX_DMA_STREAM=STM32_DMA_STREAM_ID(1,4)  STM32_SPI_SPI2_DMA_PRIORITY=2  STM32_SPI_SPI2_IRQ_PRIORITY=6  STM32_SPI_USE_SPI3=on  STM32_SPI_SPI3_RX_DMA_STREAM=STM32_DMA_STREAM_ID(1,0)  STM32_SPI_SPI3_TX_DMA_STREAM=STM32_DMA_STREAM_ID(1,7)  STM32_SPI_SPI3_DMA_PRIORITY=2  STM32_SPI_SPI3_IRQ_PRIORITY=6  STM32_SPI_DMA_ERROR_HOOK=chSysHalt()  STM32_UART_USE_USART1=off  STM32_UART_USART1_RX_DMA_STREAM=STM32_DMA_STREAM_ID(2, 5)  STM32_UART_USART1_TX_DMA_STREAM=STM32_DMA_STREAM_ID(2, 7)  STM32_UART_USART1_IRQ_PRIORITY=4  STM32_UART_USART1_DMA_PRIORITY=1  STM32_UART_USE_USART2=off  STM32_UART_USART2_RX_DMA_STREAM=STM32_DMA_STREAM_ID(1, 5)  STM32_UART_USART2_TX_DMA_STREAM=STM32_DMA_STREAM_ID(1, 6)  STM32_UART_USART2_IRQ_PRIORITY=4  STM32_UART_USART2_DMA_PRIORITY=1  STM32_UART_USE_USART3=off  STM32_UART_USART3_RX_DMA_STREAM=STM32_DMA_STREAM_ID(1, 1)  STM32_UART_USART3_TX_DMA_STREAM=STM32_DMA_STREAM_ID(1, 3)  STM32_UART_USART3_IRQ_PRIORITY=4  STM32_UART_USART3_DMA_PRIORITY=1  STM32_UART_USE_USART6=off  STM32_UART_USART6_RX_DMA_STREAM=STM32_DMA_STREAM_ID(2, 2)  STM32_UART_USART6_TX_DMA_STREAM=STM32_DMA_STREAM_ID(2, 7)  STM32_UART_USART6_IRQ_PRIORITY=4  STM32_UART_USART6_DMA_PRIORITY=1  STM32_UART_DMA_ERROR_HOOK=chSysHalt()  STM32_USB_USE_OTG1=off  STM32_USB_OTG1_IRQ_PRIORITY=2  STM32_USB_OTG1_RX_FIFO_SIZE=512  STM32_USB_USE_OTG2=off  STM32_USB_OTG2_IRQ_PRIORITY=2  STM32_USB_OTG2_RX_FIFO_SIZE=1024  STM32_USB_OTG_THREAD_PRIO=LOWPRIO  STM32_USB_OTG_THREAD_STACK_SIZE=128  STM32_USB_OTGFIFO_FILL_BASEPRI=0
  wires:
  pal_Config/1(PA0) -> Subsystem3/1(PD15), Rate Transition2/1, Rate Transition3/1
  Rate Transition3/1 -> Subsystem4/1(PD12)
  Rate Transition2/1 -> Subsystem2/1(PD13)

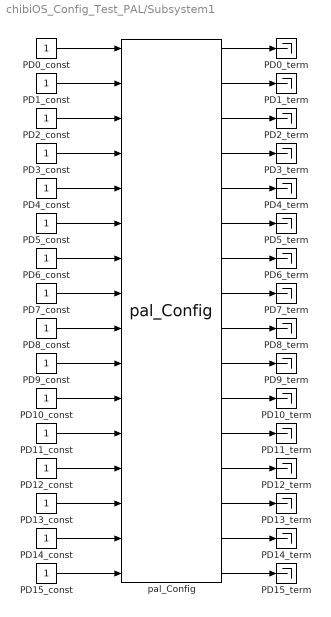
== system chibiOS_Config_Test_PAL/Subsystem1 ==
  PD0_const : Constant  OutDataTypeStr=Inherit: Inherit via back propagation
  PD0_term : Terminator
  PD10_const : Constant  OutDataTypeStr=Inherit: Inherit via back propagation
  PD10_term : Terminator
  PD11_const : Constant  OutDataTypeStr=Inherit: Inherit via back propagation
  PD11_term : Terminator
  PD12_const : Constant  OutDataTypeStr=Inherit: Inherit via back propagation
  PD12_term : Terminator
  PD13_const : Constant  OutDataTypeStr=Inherit: Inherit via back propagation
  PD13_term : Terminator
  PD14_const : Constant  OutDataTypeStr=Inherit: Inherit via back propagation
  PD14_term : Terminator
  PD15_const : Constant  OutDataTypeStr=Inherit: Inherit via back propagation
  PD15_term : Terminator
  PD1_const : Constant  OutDataTypeStr=Inherit: Inherit via back propagation
  PD1_term : Terminator
  PD2_const : Constant  OutDataTypeStr=Inherit: Inherit via back propagation
  PD2_term : Terminator
  PD3_const : Constant  OutDataTypeStr=Inherit: Inherit via back propagation
  PD3_term : Terminator
  PD4_const : Constant  OutDataTypeStr=Inherit: Inherit via back propagation
  PD4_term : Terminator
  PD5_const : Constant  OutDataTypeStr=Inherit: Inherit via back propagation
  PD5_term : Terminator
  PD6_const : Constant  OutDataTypeStr=Inherit: Inherit via back propagation
  PD6_term : Terminator
  PD7_const : Constant  OutDataTypeStr=Inherit: Inherit via back propagation
  PD7_term : Terminator
  PD8_const : Constant  OutDataTypeStr=Inherit: Inherit via back propagation
  PD8_term : Terminator
  PD9_const : Constant  OutDataTypeStr=Inherit: Inherit via back propagation
  PD9_term : Terminator
  pal_Config : M-S-Function  FunctionName=pal_Config  Parameters=portName,pin0,pin1,pin2,pin3,pin4,pin5,pin6,pin7,pin8,pin9,pin10,pin11,pin12,pin13,pin14,pin15,pal_Ts  mask(pal_Config){}
  wires:
  PD0_const/1 -> pal_Config/1
  pal_Config/1 -> PD0_term/1
  PD1_const/1 -> pal_Config/2
  pal_Config/2 -> PD1_term/1
  PD2_const/1 -> pal_Config/3
  pal_Config/3 -> PD2_term/1
  PD3_const/1 -> pal_Config/4
  pal_Config/4 -> PD3_term/1
  PD4_const/1 -> pal_Config/5
  pal_Config/5 -> PD4_term/1
  PD5_const/1 -> pal_Config/6
  pal_Config/6 -> PD5_term/1
  PD6_const/1 -> pal_Config/7
  pal_Config/7 -> PD6_term/1
  PD7_const/1 -> pal_Config/8
  pal_Config/8 -> PD7_term/1
  PD8_const/1 -> pal_Config/9
  pal_Config/9 -> PD8_term/1
  PD9_const/1 -> pal_Config/10
  pal_Config/10 -> PD9_term/1
  PD10_const/1 -> pal_Config/11
  pal_Config/11 -> PD10_term/1
  PD11_const/1 -> pal_Config/12
  pal_Config/12 -> PD11_term/1
  pal_Config/14 -> PD13_term/1
  pal_Config/15 -> PD14_term/1
  pal_Config/13 -> PD12_term/1
  pal_Config/16 -> PD15_term/1
  PD12_const/1 -> pal_Config/13
  PD13_const/1 -> pal_Config/14
  PD15_const/1 -> pal_Config/16
  PD14_const/1 -> pal_Config/15

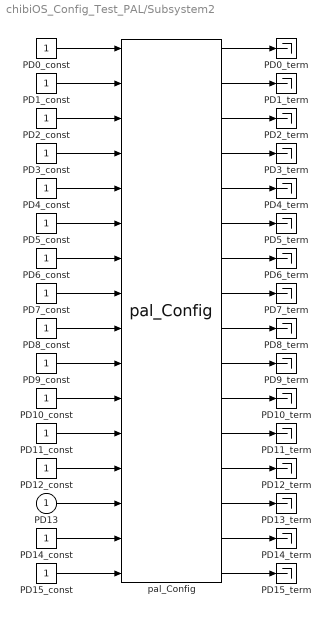
== system chibiOS_Config_Test_PAL/Subsystem2 ==
  PD13 : Inport
  PD0_const : Constant  OutDataTypeStr=Inherit: Inherit via back propagation
  PD0_term : Terminator
  PD10_const : Constant  OutDataTypeStr=Inherit: Inherit via back propagation
  PD10_term : Terminator
  PD11_const : Constant  OutDataTypeStr=Inherit: Inherit via back propagation
  PD11_term : Terminator
  PD12_const : Constant  OutDataTypeStr=Inherit: Inherit via back propagation
  PD12_term : Terminator
  PD13_term : Terminator
  PD14_const : Constant  OutDataTypeStr=Inherit: Inherit via back propagation
  PD14_term : Terminator
  PD15_const : Constant  OutDataTypeStr=Inherit: Inherit via back propagation
  PD15_term : Terminator
  PD1_const : Constant  OutDataTypeStr=Inherit: Inherit via back propagation
  PD1_term : Terminator
  PD2_const : Constant  OutDataTypeStr=Inherit: Inherit via back propagation
  PD2_term : Terminator
  PD3_const : Constant  OutDataTypeStr=Inherit: Inherit via back propagation
  PD3_term : Terminator
  PD4_const : Constant  OutDataTypeStr=Inherit: Inherit via back propagation
  PD4_term : Terminator
  PD5_const : Constant  OutDataTypeStr=Inherit: Inherit via back propagation
  PD5_term : Terminator
  PD6_const : Constant  OutDataTypeStr=Inherit: Inherit via back propagation
  PD6_term : Terminator
  PD7_const : Constant  OutDataTypeStr=Inherit: Inherit via back propagation
  PD7_term : Terminator
  PD8_const : Constant  OutDataTypeStr=Inherit: Inherit via back propagation
  PD8_term : Terminator
  PD9_const : Constant  OutDataTypeStr=Inherit: Inherit via back propagation
  PD9_term : Terminator
  pal_Config : M-S-Function  FunctionName=pal_Config  Parameters=portName,pin0,pin1,pin2,pin3,pin4,pin5,pin6,pin7,pin8,pin9,pin10,pin11,pin12,pin13,pin14,pin15,pal_Ts  mask(pal_Config){}
  wires:
  PD12_const/1 -> pal_Config/13
  PD14_const/1 -> pal_Config/15
  pal_Config/16 -> PD15_term/1
  pal_Config/13 -> PD12_term/1
  pal_Config/15 -> PD14_term/1
  pal_Config/14 -> PD13_term/1
  pal_Config/12 -> PD11_term/1
  PD11_const/1 -> pal_Config/12
  pal_Config/11 -> PD10_term/1
  PD10_const/1 -> pal_Config/11
  pal_Config/10 -> PD9_term/1
  PD9_const/1 -> pal_Config/10
  pal_Config/9 -> PD8_term/1
  PD8_const/1 -> pal_Config/9
  pal_Config/8 -> PD7_term/1
  PD7_const/1 -> pal_Config/8
  pal_Config/7 -> PD6_term/1
  PD6_const/1 -> pal_Config/7
  pal_Config/6 -> PD5_term/1
  PD5_const/1 -> pal_Config/6
  pal_Config/5 -> PD4_term/1
  PD4_const/1 -> pal_Config/5
  pal_Config/4 -> PD3_term/1
  PD3_const/1 -> pal_Config/4
  pal_Config/3 -> PD2_term/1
  PD2_const/1 -> pal_Config/3
  pal_Config/2 -> PD1_term/1
  PD1_const/1 -> pal_Config/2
  pal_Config/1 -> PD0_term/1
  PD0_const/1 -> pal_Config/1
  PD13/1 -> pal_Config/14
  PD15_const/1 -> pal_Config/16

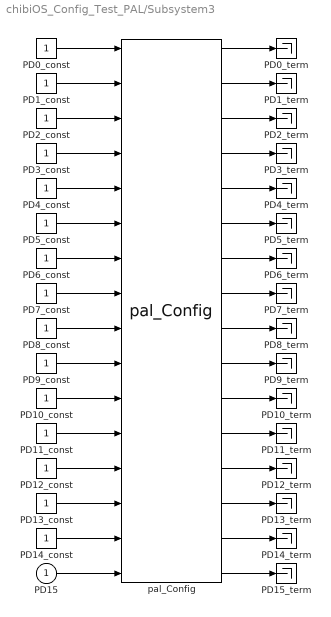
== system chibiOS_Config_Test_PAL/Subsystem3 ==
  PD15 : Inport
  PD0_const : Constant  OutDataTypeStr=Inherit: Inherit via back propagation
  PD0_term : Terminator
  PD10_const : Constant  OutDataTypeStr=Inherit: Inherit via back propagation
  PD10_term : Terminator
  PD11_const : Constant  OutDataTypeStr=Inherit: Inherit via back propagation
  PD11_term : Terminator
  PD12_const : Constant  OutDataTypeStr=Inherit: Inherit via back propagation
  PD12_term : Terminator
  PD13_const : Constant  OutDataTypeStr=Inherit: Inherit via back propagation
  PD13_term : Terminator
  PD14_const : Constant  OutDataTypeStr=Inherit: Inherit via back propagation
  PD14_term : Terminator
  PD15_term : Terminator
  PD1_const : Constant  OutDataTypeStr=Inherit: Inherit via back propagation
  PD1_term : Terminator
  PD2_const : Constant  OutDataTypeStr=Inherit: Inherit via back propagation
  PD2_term : Terminator
  PD3_const : Constant  OutDataTypeStr=Inherit: Inherit via back propagation
  PD3_term : Terminator
  PD4_const : Constant  OutDataTypeStr=Inherit: Inherit via back propagation
  PD4_term : Terminator
  PD5_const : Constant  OutDataTypeStr=Inherit: Inherit via back propagation
  PD5_term : Terminator
  PD6_const : Constant  OutDataTypeStr=Inherit: Inherit via back propagation
  PD6_term : Terminator
  PD7_const : Constant  OutDataTypeStr=Inherit: Inherit via back propagation
  PD7_term : Terminator
  PD8_const : Constant  OutDataTypeStr=Inherit: Inherit via back propagation
  PD8_term : Terminator
  PD9_const : Constant  OutDataTypeStr=Inherit: Inherit via back propagation
  PD9_term : Terminator
  pal_Config : M-S-Function  FunctionName=pal_Config  Parameters=portName,pin0,pin1,pin2,pin3,pin4,pin5,pin6,pin7,pin8,pin9,pin10,pin11,pin12,pin13,pin14,pin15,pal_Ts  mask(pal_Config){}
  wires:
  PD13_const/1 -> pal_Config/14
  PD12_const/1 -> pal_Config/13
  PD14_const/1 -> pal_Config/15
  pal_Config/16 -> PD15_term/1
  pal_Config/13 -> PD12_term/1
  pal_Config/15 -> PD14_term/1
  pal_Config/14 -> PD13_term/1
  pal_Config/12 -> PD11_term/1
  PD11_const/1 -> pal_Config/12
  pal_Config/11 -> PD10_term/1
  PD10_const/1 -> pal_Config/11
  pal_Config/10 -> PD9_term/1
  PD9_const/1 -> pal_Config/10
  pal_Config/9 -> PD8_term/1
  PD8_const/1 -> pal_Config/9
  pal_Config/8 -> PD7_term/1
  PD7_const/1 -> pal_Config/8
  pal_Config/7 -> PD6_term/1
  PD6_const/1 -> pal_Config/7
  pal_Config/6 -> PD5_term/1
  PD5_const/1 -> pal_Config/6
  pal_Config/5 -> PD4_term/1
  PD4_const/1 -> pal_Config/5
  pal_Config/4 -> PD3_term/1
  PD3_const/1 -> pal_Config/4
  pal_Config/3 -> PD2_term/1
  PD2_const/1 -> pal_Config/3
  pal_Config/2 -> PD1_term/1
  PD1_const/1 -> pal_Config/2
  pal_Config/1 -> PD0_term/1
  PD0_const/1 -> pal_Config/1
  PD15/1 -> pal_Config/16

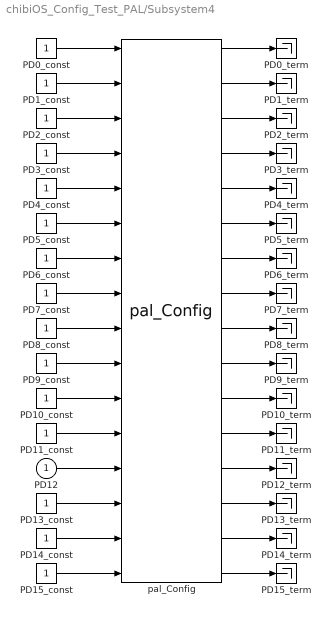
== system chibiOS_Config_Test_PAL/Subsystem4 ==
  PD12 : Inport
  PD0_const : Constant  OutDataTypeStr=Inherit: Inherit via back propagation
  PD0_term : Terminator
  PD10_const : Constant  OutDataTypeStr=Inherit: Inherit via back propagation
  PD10_term : Terminator
  PD11_const : Constant  OutDataTypeStr=Inherit: Inherit via back propagation
  PD11_term : Terminator
  PD12_term : Terminator
  PD13_const : Constant  OutDataTypeStr=Inherit: Inherit via back propagation
  PD13_term : Terminator
  PD14_const : Constant  OutDataTypeStr=Inherit: Inherit via back propagation
  PD14_term : Terminator
  PD15_const : Constant  OutDataTypeStr=Inherit: Inherit via back propagation
  PD15_term : Terminator
  PD1_const : Constant  OutDataTypeStr=Inherit: Inherit via back propagation
  PD1_term : Terminator
  PD2_const : Constant  OutDataTypeStr=Inherit: Inherit via back propagation
  PD2_term : Terminator
  PD3_const : Constant  OutDataTypeStr=Inherit: Inherit via back propagation
  PD3_term : Terminator
  PD4_const : Constant  OutDataTypeStr=Inherit: Inherit via back propagation
  PD4_term : Terminator
  PD5_const : Constant  OutDataTypeStr=Inherit: Inherit via back propagation
  PD5_term : Terminator
  PD6_const : Constant  OutDataTypeStr=Inherit: Inherit via back propagation
  PD6_term : Terminator
  PD7_const : Constant  OutDataTypeStr=Inherit: Inherit via back propagation
  PD7_term : Terminator
  PD8_const : Constant  OutDataTypeStr=Inherit: Inherit via back propagation
  PD8_term : Terminator
  PD9_const : Constant  OutDataTypeStr=Inherit: Inherit via back propagation
  PD9_term : Terminator
  pal_Config : M-S-Function  FunctionName=pal_Config  Parameters=portName,pin0,pin1,pin2,pin3,pin4,pin5,pin6,pin7,pin8,pin9,pin10,pin11,pin12,pin13,pin14,pin15,pal_Ts  mask(pal_Config){}
  wires:
  PD0_const/1 -> pal_Config/1
  pal_Config/1 -> PD0_term/1
  PD1_const/1 -> pal_Config/2
  pal_Config/2 -> PD1_term/1
  PD2_const/1 -> pal_Config/3
  pal_Config/3 -> PD2_term/1
  PD3_const/1 -> pal_Config/4
  pal_Config/4 -> PD3_term/1
  PD4_const/1 -> pal_Config/5
  pal_Config/5 -> PD4_term/1
  PD5_const/1 -> pal_Config/6
  pal_Config/6 -> PD5_term/1
  PD6_const/1 -> pal_Config/7
  pal_Config/7 -> PD6_term/1
  PD7_const/1 -> pal_Config/8
  pal_Config/8 -> PD7_term/1
  PD8_const/1 -> pal_Config/9
  pal_Config/9 -> PD8_term/1
  PD9_const/1 -> pal_Config/10
  pal_Config/10 -> PD9_term/1
  PD10_const/1 -> pal_Config/11
  pal_Config/11 -> PD10_term/1
  PD11_const/1 -> pal_Config/12
  pal_Config/12 -> PD11_term/1
  pal_Config/14 -> PD13_term/1
  pal_Config/15 -> PD14_term/1
  pal_Config/13 -> PD12_term/1
  pal_Config/16 -> PD15_term/1
  PD13_const/1 -> pal_Config/14
  PD15_const/1 -> pal_Config/16
  PD14_const/1 -> pal_Config/15
  PD12/1 -> pal_Config/13

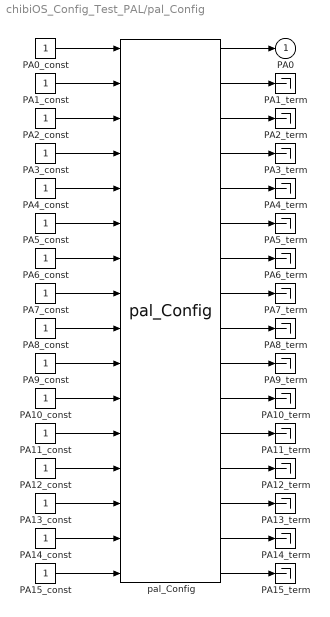
== system chibiOS_Config_Test_PAL/pal_Config ==
  PA0_const : Constant  OutDataTypeStr=Inherit: Inherit via back propagation
  PA10_const : Constant  OutDataTypeStr=Inherit: Inherit via back propagation
  PA10_term : Terminator
  PA11_const : Constant  OutDataTypeStr=Inherit: Inherit via back propagation
  PA11_term : Terminator
  PA12_const : Constant  OutDataTypeStr=Inherit: Inherit via back propagation
  PA12_term : Terminator
  PA13_const : Constant  OutDataTypeStr=Inherit: Inherit via back propagation
  PA13_term : Terminator
  PA14_const : Constant  OutDataTypeStr=Inherit: Inherit via back propagation
  PA14_term : Terminator
  PA15_const : Constant  OutDataTypeStr=Inherit: Inherit via back propagation
  PA15_term : Terminator
  PA1_const : Constant  OutDataTypeStr=Inherit: Inherit via back propagation
  PA1_term : Terminator
  PA2_const : Constant  OutDataTypeStr=Inherit: Inherit via back propagation
  PA2_term : Terminator
  PA3_const : Constant  OutDataTypeStr=Inherit: Inherit via back propagation
  PA3_term : Terminator
  PA4_const : Constant  OutDataTypeStr=Inherit: Inherit via back propagation
  PA4_term : Terminator
  PA5_const : Constant  OutDataTypeStr=Inherit: Inherit via back propagation
  PA5_term : Terminator
  PA6_const : Constant  OutDataTypeStr=Inherit: Inherit via back propagation
  PA6_term : Terminator
  PA7_const : Constant  OutDataTypeStr=Inherit: Inherit via back propagation
  PA7_term : Terminator
  PA8_const : Constant  OutDataTypeStr=Inherit: Inherit via back propagation
  PA8_term : Terminator
  PA9_const : Constant  OutDataTypeStr=Inherit: Inherit via back propagation
  PA9_term : Terminator
  pal_Config : M-S-Function  FunctionName=pal_Config  Parameters=portName,pin0,pin1,pin2,pin3,pin4,pin5,pin6,pin7,pin8,pin9,pin10,pin11,pin12,pin13,pin14,pin15,pal_Ts  mask(pal_Config){}
  PA0 : Outport
  wires:
  pal_Config/2 -> PA1_term/1
  PA0_const/1 -> pal_Config/1
  PA2_const/1 -> pal_Config/3
  pal_Config/3 -> PA2_term/1
  PA3_const/1 -> pal_Config/4
  pal_Config/4 -> PA3_term/1
  PA4_const/1 -> pal_Config/5
  pal_Config/5 -> PA4_term/1
  PA5_const/1 -> pal_Config/6
  pal_Config/6 -> PA5_term/1
  PA6_const/1 -> pal_Config/7
  pal_Config/7 -> PA6_term/1
  PA7_const/1 -> pal_Config/8
  pal_Config/8 -> PA7_term/1
  PA8_const/1 -> pal_Config/9
  pal_Config/9 -> PA8_term/1
  PA9_const/1 -> pal_Config/10
  pal_Config/10 -> PA9_term/1
  PA10_const/1 -> pal_Config/11
  pal_Config/11 -> PA10_term/1
  PA11_const/1 -> pal_Config/12
  pal_Config/12 -> PA11_term/1
  PA12_const/1 -> pal_Config/13
  pal_Config/13 -> PA12_term/1
  PA13_const/1 -> pal_Config/14
  pal_Config/14 -> PA13_term/1
  PA14_const/1 -> pal_Config/15
  pal_Config/15 -> PA14_term/1
  PA15_const/1 -> pal_Config/16
  pal_Config/16 -> PA15_term/1
  pal_Config/1 -> PA0/1
  PA1_const/1 -> pal_Config/2
